simulink model "simu_Blanca2023"  (R2023b)
settings: Solver=VariableStepAuto  StartTime=0.0  StopTime=Tsim  RelTol=1e-3
values from neighbouring files (symbols this model uses):
  A_o = [1, tau*(1 - a), tau*Ts - tau^2*(1 - a) ... (first row only)    [Blanca2023.m]
  b0 = 4.5    [Blanca2023.m]
  B_o = b0 * [tau*Ts - tau^2*(1 - a) ... (first row only)    [Blanca2023.m]
  C_o = [1, 0, 0]    [Blanca2023.m]
  dist = 1    [Blanca2023.m]
  du_max = 1    [Blanca2023.m]    (also in Blanca2023_solver.m = block.DialogPrm(10).Data)
  du_min = -1    [Blanca2023.m]    (also in Blanca2023_solver.m = block.DialogPrm(11).Data)
  G = zeros(N,Nu)    [Blanca2023.m]    (also in Blanca2023_solver.m = block.DialogPrm(15).Data)
  G_eq = zeros(n_eq, Nu)    [Blanca2023.m]    (also in Blanca2023_solver.m = block.DialogPrm(5).Data)
  gamma = 0.001    [Blanca2023.m]    (also in Blanca2023_solver.m = block.DialogPrm(16).Data)
  H_aug = blkdiag(H_du, 2 * eps_2 * eye(n_eq))    [Blanca2023.m]    (also in Blanca2023_solver.m = block.DialogPrm(12).Data)
  L_o = [lo1; lo2; lo3]    [Blanca2023.m]
  N = 85    [Blanca2023.m]    (also in Blanca2023_solver.m = block.DialogPrm(1).Data)
  n_eq = 2    [Blanca2023.m]    (also in Blanca2023_solver.m = block.DialogPrm(13).Data)
  Nu = 20    [Blanca2023.m]    (also in Blanca2023_solver.m = block.DialogPrm(2).Data)
  P = zeros(N,2)    [Blanca2023.m]    (also in Blanca2023_solver.m = block.DialogPrm(3).Data)
  P_eq = zeros(n_eq, 2)    [Blanca2023.m]    (also in Blanca2023_solver.m = block.DialogPrm(6).Data)
  T_dist = 15    [Blanca2023.m]
  Ts = 0.1    [Blanca2023.m]    (also in Blanca2023_solver.m = block.DialogPrm(14).Data)
  u_max = 5    [Blanca2023.m]    (also in Blanca2023_solver.m = block.DialogPrm(8).Data)
  u_min = -5    [Blanca2023.m]    (also in Blanca2023_solver.m = block.DialogPrm(9).Data)
  V_B = zeros(N,1)    [Blanca2023.m]    (also in Blanca2023_solver.m = block.DialogPrm(4).Data)
  V_B_eq = zeros(n_eq, 1)    [Blanca2023.m]    (also in Blanca2023_solver.m = block.DialogPrm(7).Data)
undefined symbols (not defined in the file or in its folder): A_p, B_p, C_p, D_p, simulation
settings Model: Creator=sergio  LastModifiedBy=sergio

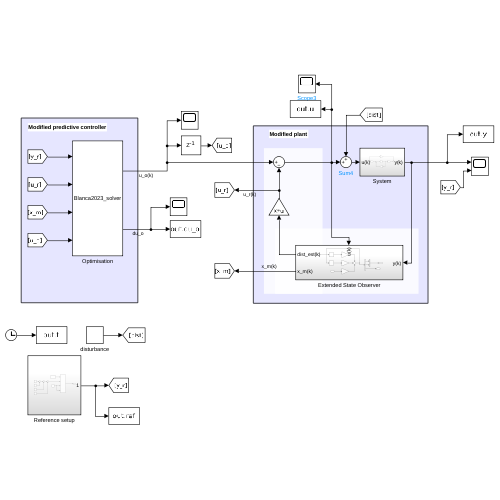
[thumbnail: Simulink's stored preview of the top-level diagram]
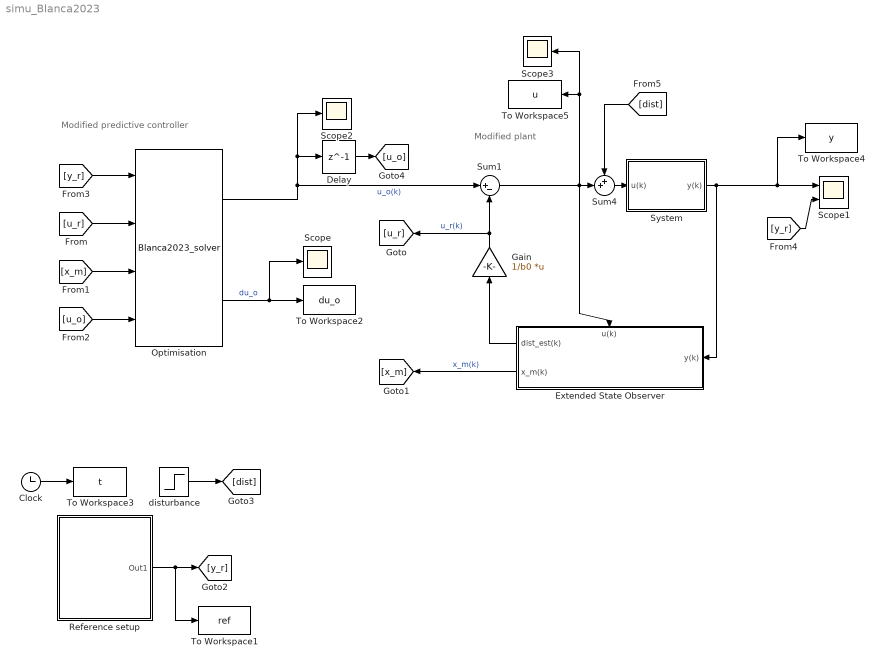
== system simu_Blanca2023 ==
  note: Modified predictive controller
  note: Modified plant
  Clock : Clock
  Delay : Delay  DelayLength=1  SampleTime=Ts
  Extended State Observer : Subsystem
      settings: PortSchema="{\"entries\":[{\"content\":{\"sides\":[{\"content\":{\"connectorIds\":[\"In1\"]},\"type\":\"ConnectorPlacement.EquallySpacedRectSide\",\"uuid\":\"cd176947-fcfb-4df2-a5a8-2468070b6871\"},{\"content\":{\"connectorIds\":[\"Out1\",\"Out2\"],\"side\":\"RIGHT\"},\"type\":\"ConnectorPlacement.EquallySpacedRectSide\",\"uuid\":\"6b898551-d171-49d4-aa03-7a53cde05bfa\"},{\"content\":{\"connectorIds\":[\"In2\"],\"side\":\"TOP\"},\"type\":\"ConnectorPlacement.EquallySpacedRectSide\",\"uuid\":\"e7f80a75-22d0-47e7-b029-4dc656fe7605\"}]},\"type\":\"ConnectorPlacement.EquallySpacedConnector\",\"uuid\":\"3f93b126-fd73-4b26-b8bd-256c731d55c9\"}],\"packageUris\":[\"http://schema.mathworks.com/mf0/Connector/R2020b\"],\"version\":\"1.0\"}"
  Gain : Gain  Gain=1/b0  Multiplication=Matrix(K*u)
  Optimisation : M-S-Function  FunctionName=Blanca2023_solver  Parameters=N,Nu,P,V_B,G_eq,P_eq,V_B_eq,u_max,u_min,du_max,du_min,H_aug,n_eq,Ts,G,gamma
  Reference setup : Subsystem
  Scope : Scope
  Scope1 : Scope  NumInputPorts=2
  Scope2 : Scope
  Scope3 : Scope
  Sum1 : Sum  Inputs=|+-
  Sum4 : Sum  Inputs=++|
  System : Subsystem
  To Workspace1 : ToWorkspace  VariableName=ref  SampleTime=Ts
      settings: Save2DSignal=2-D array (concatenate along first dimension)
  To Workspace2 : ToWorkspace  VariableName=du_o  SampleTime=Ts
      settings: Save2DSignal=2-D array (concatenate along first dimension)
  To Workspace3 : ToWorkspace  VariableName=t  SampleTime=Ts
      settings: Save2DSignal=2-D array (concatenate along first dimension)
  To Workspace4 : ToWorkspace  VariableName=y  SampleTime=Ts
      settings: Save2DSignal=2-D array (concatenate along first dimension)
  To Workspace5 : ToWorkspace  VariableName=u  SampleTime=Ts
      settings: Save2DSignal=2-D array (concatenate along first dimension)
  disturbance : Step  Time=T_dist  After=dist  SampleTime=Ts
  wires:
  Clock/1 -> To Workspace3/1
  System/1(y(k)) -> To Workspace4/1, Scope1/1, Extended State Observer/1(y(k))
  Gain/1 -> Sum1/2, [u_r]  "u_r(k)"
  Extended State Observer/1(dist_est(k)) -> Gain/1
  Optimisation/1 -> Scope2/1, Delay/1, Sum1/1  "u_o(k)"
  Extended State Observer/2(x_m(k)) -> [x_m]  "x_m(k)"
  [y_r] -> Optimisation/1
  [u_r] -> Optimisation/2
  [x_m] -> Optimisation/3
  Delay/1 -> [u_o]
  [u_o] -> Optimisation/4
  Optimisation/2 -> To Workspace2/1, Scope/1  "du_o"
  [y_r] -> Scope1/2
  Sum4/1 -> System/1(u(k))
  Sum1/1 -> Extended State Observer/2(u(k)), To Workspace5/1, Scope3/1, Sum4/2
  [dist] -> Sum4/1
  Reference setup/1(Out1) -> To Workspace1/1, [y_r]
  disturbance/1 -> [dist]

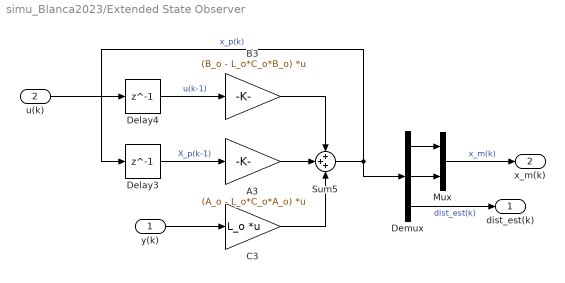
== system simu_Blanca2023/Extended State Observer ==
  y(k) : Inport
  u(k) : Inport  Port=2
  A3 : Gain  Gain=(A_o - L_o*C_o*A_o)  Multiplication=Matrix(K*u)
  B3 : Gain  Gain=(B_o - L_o*C_o*B_o)  Multiplication=Matrix(K*u)
  C3 : Gain  Gain=L_o  Multiplication=Matrix(K*u)
  Delay3 : Delay  DelayLength=1  SampleTime=Ts
  Delay4 : Delay  DelayLength=1  SampleTime=Ts
  Demux : Demux  Outputs=3
  Mux : Mux  Inputs=2
  Sum5 : Sum  Inputs=+++
  dist_est(k) : Outport
  x_m(k) : Outport  Port=2
  wires:
  Delay3/1 -> A3/1  "X_p(k-1)"
  Demux/3 -> dist_est(k)/1  "dist_est(k)"
  A3/1 -> Sum5/2
  y(k)/1 -> C3/1
  Demux/1 -> Mux/1
  u(k)/1 -> Delay4/1
  Demux/2 -> Mux/2
  Sum5/1 -> Demux/1, Delay3/1  "x_p(k)"
  Delay4/1 -> B3/1  "u(k-1)"
  B3/1 -> Sum5/1
  Mux/1 -> x_m(k)/1  "x_m(k)"
  C3/1 -> Sum5/3

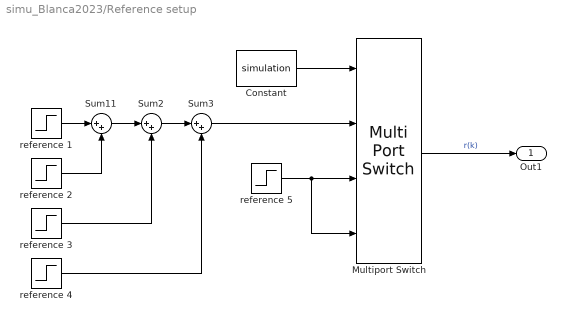
== system simu_Blanca2023/Reference setup ==
  Constant : Constant  Value=simulation
  Multiport Switch : MultiPortSwitch  SaturateOnIntegerOverflow=off  InputSameDT=off
  Sum11 : Sum  Inputs=|++
  Sum2 : Sum  Inputs=|++
  Sum3 : Sum  Inputs=|++
  reference 1 : Step  Time=0  After=15  SampleTime=Ts
  reference 2 : Step  Time=4  After=30  SampleTime=Ts
  reference 3 : Step  Time=10  After=-15  SampleTime=Ts
  reference 4 : Step  Time=16  After=-10  SampleTime=Ts
  reference 5 : Step  Time=0  SampleTime=Ts
  Out1 : Outport
  wires:
  Constant/1 -> Multiport Switch/1
  Sum3/1 -> Multiport Switch/2
  reference 2/1 -> Sum11/2
  Sum11/1 -> Sum2/1
  reference 4/1 -> Sum3/2
  reference 5/1 -> Multiport Switch/4, Multiport Switch/3
  Multiport Switch/1 -> Out1/1  "r(k)"
  reference 3/1 -> Sum2/2
  reference 1/1 -> Sum11/1
  Sum2/1 -> Sum3/1

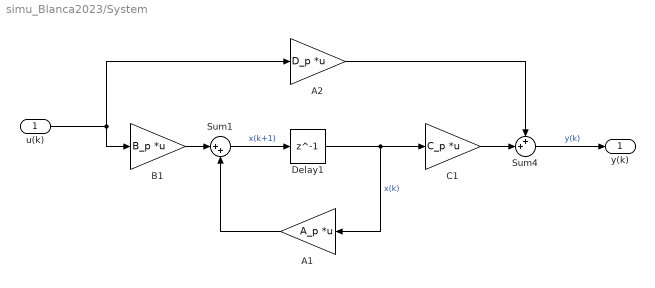
== system simu_Blanca2023/System ==
  u(k) : Inport
  A1 : Gain  Gain=A_p  Multiplication=Matrix(K*u)
  A2 : Gain  Gain=D_p  Multiplication=Matrix(K*u)
  B1 : Gain  Gain=B_p  Multiplication=Matrix(K*u)
  C1 : Gain  Gain=C_p  Multiplication=Matrix(K*u)
  Delay1 : Delay  DelayLength=1  SampleTime=Ts
  Sum1 : Sum  Inputs=|++
  Sum4 : Sum  Inputs=++|
  y(k) : Outport
  wires:
  A1/1 -> Sum1/2
  u(k)/1 -> B1/1, A2/1
  A2/1 -> Sum4/1
  Delay1/1 -> A1/1, C1/1  "x(k)"
  C1/1 -> Sum4/2
  Sum1/1 -> Delay1/1  "x(k+1)"
  B1/1 -> Sum1/1
  Sum4/1 -> y(k)/1  "y(k)"
